simulink model "TutorialVariants"
settings: Solver=ode1  StartTime=0.0  StopTime=Inf  FixedStep=0.001  RelTol=1e-3
PostLoadFcn:
  | , if any(exist('dsrtsu_mdlpostloadfcn', 'file') == [2, 3, 6]), try dsrtsu_mdlpostloadfcn('Execute', bdroot); catch fprintf('Error in PostLoadFcn (dsrtsu_mdlpostloadfcn) for model "%s":\n %s\n', bdroot, lasterr); end, end,
undefined symbols (not defined in the file): rticanmm_blockfcn, rticanmm_initfcn
libraries: rtimmsu_dsrtlib x4
settings Model: RTICANMMDATA=struct('GeneralSetupData',struct('modelroot','E:\projects\dSPACE-RLS-Variants\current\RTICANMM\Components\Tutorial\Lesson10_results\RTICANMMTutorial_Lesson10','generalsettings',struct('filesettings',struct('destfolder',struct('Name','RTICANMM_FILES','Check',1),'buildfolder',struct('Name','.','Check',1),'AbsDestfolder',struct('Name','E:\projects\dSPACE-RLS-Variants\current\RTICANMM\Components\Tutorial\Lesson10_results\RTICANMMTutorial_Lesson10\RTICANMM_FILES'),'AbsBuildfolder',struct('Name','E:\projects\dSPACE-RLS-Variants\current\RTICANMM\Components\Tutorial\Lesson10_results\RTICANMMTutorial_Lesson10'))),'options',struct('addpaths',1,'rmpaths',1,'addtrcexclusion',logical(1),'cannavigator',struct('checkmonitoring',0,'checkinternmonitoring',1,'serviceno','31','hostservicedefheader',struct('name','RTICANMMHostService_TutorialVariants.h','path',['E:\CANMM_Tutorial\RLS2008-A\aus MKS\Lesson10_results\RTICANMMTutorial_Lesson10\RTICANMM_FILES\RTICANMMHostService_TutorialVariants.h'])),'show_usrtrc',0,'use_usrtrc',0,'addpath2usrmk',1),'advanced',struct('options',[1 1 1 1 1 1 1 1 1 1 1 1 1 1 1 1 1 1 1 1 1 1 1 1 1 1 1 1 1 1 1 1 1 1 1 1 1 1 1 1 1 1 1 1 1 1 1 1 1 1 1 1 1 1 1 1 1 1 1 1 1 1 1 1 1 1 1 1 1 1 1 1 1 1 1 1 1 1 1 1 1 1 1 1 1 1 1 1 1 1 1 1 1 1 1 1 1 1 1 1]),'MPSetup',{{}},'modelname','Lesson10_TutorialVariants','blockdata',struct('generalsettings',struct('filesettings',struct('destfolder',struct('Name','.','Check',1),'AbsDestfolder',struct('Name','T:\TOOL_SOURCES\CANnedy\m'),'buildfolder',struct('Name','.','Check',1),'AbsBuildfolder',struct('Name','C:\MATLAB6p5\work'))),'options',struct('addpaths',1,'rmpaths',1,'addpath2usrmk',1),'modelname','rticanmmlib','modelroot','T:\TOOL_SOURCES\CANnedy\m'),'userdata',struct('CANMMName',{{'TutVar_M1_V1','TutVar_M2','TutVar_M1_V2'}},'HostServiceChannelID',{{'TutVar_C1','TutVar_C2'}}),'RTI',struct('Type','RTI1005','Ver','7.1','Date','02-Nov-2013'),'version','3.0.735627.5512384259','MMType','RTICANMM','block',['Lesson10_TutorialVariants/RTICANMM' char(10) 'GeneralSetup']),'BuildData',struct('GeneralSetupData',struct('modelroot','D:\projects\dSPACE-RLS-Variants\current\RTICANMM\Components\Tutorial\Lesson10_results\RTICANMMTutorial_Lesson10','generalsettings',struct('filesettings',struct('destfolder',struct('Name','RTICANMM_FILES','Check',1),'buildfolder',struct('Name','.','Check',1),'AbsDestfolder',struct('Name','D:\projects\dSPACE-RLS-Variants\current\RTICANMM\Components\Tutorial\Lesson10_results\RTICANMMTutorial_Lesson10\RTICANMM_FILES'),'AbsBuildfolder',struct('Name','D:\projects\dSPACE-RLS-Variants\current\RTICANMM\Components\Tutorial\Lesson10_results\RTICANMMTutorial_Lesson10'))),'options',struct('addpaths',1,'rmpaths',1,'addtrcexclusion',logical(1),'cannavigator',struct('checkmonitoring',0,'checkinternmonitoring',1,'serviceno','31','hostservicedefheader',struct('name','RTICANMMHostService_TutorialVariants.h','path',['E:\CANMM_Tutorial\RLS2008-A\aus MKS\Lesson10_results\RTICANMMTutorial_Lesson10\RTICANMM_FILES\RTICANMMHostService_TutorialVariants.h'])),'show_usrtrc',0,'use_usrtrc',0,'addpath2usrmk',1),'advanced',struct('options',[1 1 1 1 1 1 1 1 1 1 1 1 1 1 1 1 1 1 1 1 1 1 1 1 1 1 1 1 1 1 1 1 1 1 1 1 1 1 1 1 1 1 1 1 1 1 1 1 1 1 1 1 1 1 1 1 1 1 1 1 1 1 1 1 1 1 1 1 1 1 1 1 1 1 1 1 1 1 1 1 1 1 1 1 1 1 1 1 1 1 1 1 1 1 1 1 1 1 1 1]),'MPSetup',{{}},'modelname','Lesson10_TutorialVariants','blockdata',struct('generalsettings',struct('filesettings',struct('destfolder',struct('Name','.','Check',1),'AbsDestfolder',struct('Name','T:\TOOL_SOURCES\CANnedy\m'),'buildfolder',struct('Name','.','Check',1),'AbsBuildfolder',struct('Name','C:\MATLAB6p5\work'))),'options',struct('addpaths',1,'rmpaths',1,'addpath2usrmk',1),'modelname','rticanmmlib','modelroot','T:\TOOL_SOURCES\CANnedy\m'),'userdata',struct('CANMMName',{{'TutVar_M1_V1','TutVar_M2','TutVar_M1_V2'}},'HostServiceChannelID',{{'TutVar_C1','TutVar_C2'}}),'RTI',struct('Type','RTI1005','Ver','6.6','Date','29-Nov-2010'),'version','2.5.4.734704.7639','MMType','RTICANMM','block',['Lesson10_TutorialVariants/RTICANMM' char(10) 'GeneralSetup']),'ModelBuildIsUpToDate',0))  RTILINMMDATA=struct('GeneralSetupData',[])  DSRTSU_INTERNAL_RTI_VER=430  DSRTSU_INTERNAL_RTI_TYPE=rti1005  DSRTSU_INTERNAL_RTIFLEXRAYCONFIG=60  DSRTSU_INTERNAL_RTIFPGA=30  BufferReuse=off  Creator=dSPACE GmbH  LastModifiedBy=dSPACE GmbH
settings DataIOCC: LimitDataPoints=on  SaveFormat=Array  SignalLoggingSaveFormat=ModelDataLogs  ReturnWorkspaceOutputs=off
settings OptimizationCC: BlockReduction=off  OptimizeBlockIOStorage=off  BufferReuse=off  ExpressionFolding=off  ExpressionDepthLimit=2147483647  LocalBlockOutputs=off  InitFltsAndDblsToZero=on  LifeSpan=inf  SimCompilerOptimization=Off
settings DebuggingCC: SaveWithParameterizedLinksMsg=none  UnderspecifiedInitializationDetection=Classic  MergeDetectMultiDrivingBlocksExec=none  SolverPrmCheckMsg=warning  MultiTaskCondExecSysMsg=none  FcnCallInpInsideContextMsg=Use local settings  FrameProcessingCompatibilityMsg=warning  StateNameClashWarn=warning  SFUnexpectedBacktrackingDiag=warning  SFNoUnconditionalDefaultTransitionDiag=warning
settings HardwareCC: ProdBitPerPointer=32  ProdLargestAtomicFloat=None  ProdEndianess=BigEndian  ProdWordSize=32  ProdHWDeviceType=Generic->Custom  TargetIntDivRoundTo=Zero  TargetEndianess=BigEndian  TargetHWDeviceType=Generic->Custom
settings ModelReferenceCC: PropagateSignalLabelsOutOfModel=off
settings SFSimCC: SimUseLocalCustomCode=off
settings RTWCC: SystemTargetFile=rti1005.tlc  MakeCommand=make_rti  TemplateMakefile=rti1005.tmf  Description=dSPACE DS1005 Hardware Platform  ProcessScript=rti1005_make_rtw_hook  RTWUseLocalCustomCode=off  IncludeERTFirstTime=on  RTWCompilerOptimization=Off
settings CodeAppCC: CustomSymbolStrType=$N$R$M
settings STFCustomTargetCC: TargetFcnLib=ansi_tfl_tmw.mat  CodeReplacementLibrary=ANSI_C  ParMdlRefBuildCompliant=on  GeneratePreprocessorConditionals=Disable all  SystemTargetFile=rti1005.tlc
settings GRTTargetCC: TargetFcnLib=ansi_tfl_tmw.mat  CodeReplacementLibrary=ANSI_C  CompOptLevelCompliant=off  ConcurrentExecutionCompliant=off  GeneratePreprocessorConditionals=Disable all  CombineOutputUpdateFcns=off  MatFileLogging=off  CPPClassGenCompliant=off  GRTInterface=on  ExtModeMexFile=noextcomm

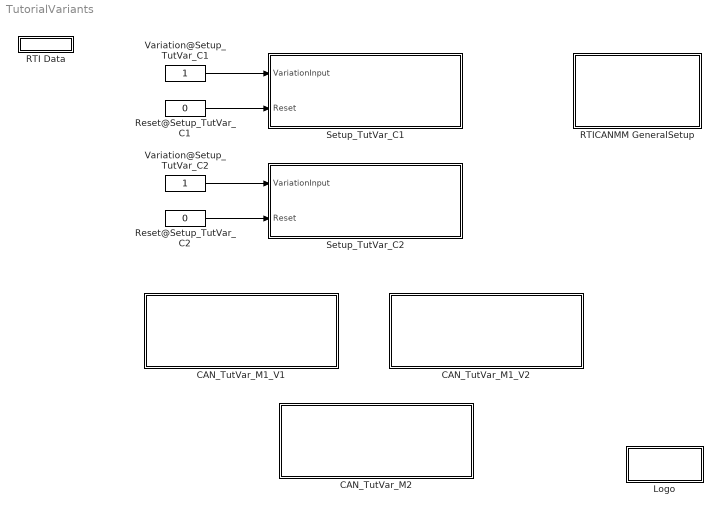
== system TutorialVariants ==
  CAN_TutVar_M1_V1 : Subsystem  InitFcn=rticanmm_blockfcn('InitFcn', 'CANnedy', gcb)  ClipboardFcn=rticanmm_blockfcn('ClipboardFcn', 'CANnedy', gcb)  mask(RTICANMM){DSProperties=struct('RTI',struct('Version',uint32(1),'BlockType',struct('isSLSource',uint8(1),'isSLSink',uint8(1),'isHWSource',uint8(0),'isHWSink',uint8(0),'isSetup',uint8(0),'isInline',uint8(1),'isNonInline',uint8(0),'isInterrupt',uint8(0),'isChannelwise',uint8(0)),'IOBoardType','RTICANMM','UnitType','RTICANMM','Identifier','Mainblock','DialogType','SL','BlockSet','RTICANMM','SlaveProcessor','CAN')), CANMMProperties=struct('RTICANMMVersion','3.0','RTICANMMVersionIntern','3.0.735627.5512384259','RTICANMMDate','02-May-2014','Settings','RTICANMM_MAIN_TutVar_M1_V1','UserTracePath','','ModelPath','E:\\projects\\dSPACE-RLS-Variants\\current\\RTICANMM\\Components\\Tutorial\\Lesson10_results\\RTICANMMTutorial_Lesson10','filesettings',struct('FileName','chassis.dbc','IsRelative',1,'ClusterId',1,'ClusterList',{{'default'}},'destfolder',struct('Name','RTICANMM_FILES','Check',1),'buildfolder',struct('Name','.','Check',1),'onlyfreerawcapture',0,'overlapping2variant',0),'onlyfreerawcapture',0,'Board','DS4302','BoardNum','1','ChannelNum','1','Variation','1','SetupId','TutVar_C1','MARK',['55E03A74395B53F8DB43BA9618B512';'A23C9334B1324361A95E8FCD407A20';'098F83A39FCF2835CF252EEA455F34';'6393CC0945E19D10F98F8B4C582B6C';'4BC1A51935C111E55014785F64462B'],'date','03-Feb-2014','clock',['03.02.2014 15:34:55'],'recreate',0,'RTIVER','RTI1005','j1939',0,'TRC',struct('include',1),'rtsupport',struct('XMLFile','E:\\projects\\dSPACE-RLS-Variants\\current\\RTICANMM\\Components\\Tutorial\\Lesson10_results\\RTICANMMTutorial_Lesson10\\RTICANMM_FILES\\RTICANMM_MAIN_TutVar_M1_V1.xml','DBCXML',struct('Path','E:\\projects\\dSPACE-RLS-Variants\\current\\RTICANMM\\Components\\Tutorial\\Lesson10_results\\RTICANMMTutorial_Lesson10\\RTICANMM_FILES\\RTICANMM_MAIN_TutVar_M1_V1_dbc.xml','support',1,'Name','chassis.dbc','Date',['09-Okt-2007 15:20:29'],'Type','mixed','DBCSupport','ON'))), CANMMType=CANnedy, CANMMUserTraceMerged=off, CANMMUserTracePath=, CANMMChannelNum=1, CANMMBoardNum=1, CANMMDestFolder=RTICANMM_FILES, CANMMFolder=., CANMMSetupId=TutVar_C1, CANMMsave2mat=['55E03A74395B53F8DB43BA9618B512';'A23C9334B1324361A95E8FCD407A20';'098F83A39FCF2835CF252EEA455F34';'6393CC0945E19D10F98F8B4C582B6C';'4BC1A51935C111E55014785F64462B'], CANMMName=TutVar_M1_V1, CANMMSettings=RTICANMM_MAIN_TutVar_M1_V1, CANMMIntermediateTag=RTICANMM_MAIN_TutVar_M1_V1_intermediate, CANMMsfcnname=RTICANMM_MAIN_TutVar_M1_V1}
      mask init:
      | rticanmm_initfcn(gcb, CANMMType, CANMMsfcnname)
      settings: AttributesFormatString=TutVar_C1[TutVar_M1_V1]: DS4302_B1_C1_V1  CopyFcn=rticanmm_blockfcn('CopyFcn', 'CANnedy', gcb)  DeleteFcn=rticanmm_blockfcn('DeleteFcn', 'CANnedy', gcb)  ModelCloseFcn=rticanmm_blockfcn('ModelCloseFcn', 'CANnedy', gcb)  NameChangeFcn=rticanmm_blockfcn('NameChangeFcn', 'CANnedy', gcb)  OpenFcn=try, rticanmm_main_gui('create',gcb); ; catch,errordlg({lasterr, '','Please check your RTI installation.'},['Error: ' upper(bdroot)], 'replace'); end  MoveFcn=rticanmm_blockfcn('MoveFcn', 'CANnedy', gcb)
      mask Help: eval('rticanmm_quickstart(''create'', gcb);', 'disp(lasterr);')
      mask Display: disp(sprintf('RTI CAN\nMultiMessage\nMainSetup'))
  CAN_TutVar_M1_V2 : Subsystem  InitFcn=rticanmm_blockfcn('InitFcn', 'CANnedy', gcb)  ClipboardFcn=rticanmm_blockfcn('ClipboardFcn', 'CANnedy', gcb)  mask(RTICANMM){DSProperties=struct('RTI',struct('Version',uint32(1),'BlockType',struct('isSLSource',uint8(1),'isSLSink',uint8(1),'isHWSource',uint8(0),'isHWSink',uint8(0),'isSetup',uint8(0),'isInline',uint8(1),'isNonInline',uint8(0),'isInterrupt',uint8(0),'isChannelwise',uint8(0)),'IOBoardType','RTICANMM','UnitType','RTICANMM','Identifier','Mainblock','DialogType','SL','BlockSet','RTICANMM','SlaveProcessor','CAN')), CANMMProperties=struct('RTICANMMVersion','3.0','RTICANMMVersionIntern','3.0.735627.5512384259','RTICANMMDate','02-May-2014','Settings','RTICANMM_MAIN_TutVar_M1_V2','UserTracePath','','ModelPath','E:\\projects\\dSPACE-RLS-Variants\\current\\RTICANMM\\Components\\Tutorial\\Lesson10_results\\RTICANMMTutorial_Lesson10','filesettings',struct('FileName','chassis_changed.dbc','IsRelative',1,'ClusterId',1,'ClusterList',{{'default'}},'destfolder',struct('Name','RTICANMM_FILES','Check',1),'buildfolder',struct('Name','.','Check',1),'onlyfreerawcapture',0,'overlapping2variant',0),'onlyfreerawcapture',0,'Board','DS4302','BoardNum','1','ChannelNum','1','Variation','2','SetupId','TutVar_C1','MARK',['7A753A0F068D0B04F07F060F8EC5AA';'9C128822ED17A9DECB1FCC6137CCCA';'527E1118F9B5998B502C4CF14A4AA0';'A533E42B0DF5453AD15DD1DE46811D';'0291723C433049D43F83E639655517'],'date','03-Feb-2014','clock',['03.02.2014 15:35:12'],'recreate',0,'RTIVER','RTI1005','j1939',0,'TRC',struct('include',1),'rtsupport',struct('XMLFile','E:\\projects\\dSPACE-RLS-Variants\\current\\RTICANMM\\Components\\Tutorial\\Lesson10_results\\RTICANMMTutorial_Lesson10\\RTICANMM_FILES\\RTICANMM_MAIN_TutVar_M1_V2.xml','DBCXML',struct('Path','E:\\projects\\dSPACE-RLS-Variants\\current\\RTICANMM\\Components\\Tutorial\\Lesson10_results\\RTICANMMTutorial_Lesson10\\RTICANMM_FILES\\RTICANMM_MAIN_TutVar_M1_V2_dbc.xml','support',1,'Name','chassis_changed.dbc','Date',['31-Mrz-2008 17:23:12'],'Type','mixed','DBCSupport','ON'))), CANMMType=CANnedy, CANMMUserTraceMerged=off, CANMMUserTracePath=, CANMMChannelNum=1, CANMMBoardNum=1, CANMMDestFolder=RTICANMM_FILES, CANMMFolder=., CANMMSetupId=TutVar_C1, CANMMsave2mat=['7A753A0F068D0B04F07F060F8EC5AA';'9C128822ED17A9DECB1FCC6137CCCA';'527E1118F9B5998B502C4CF14A4AA0';'A533E42B0DF5453AD15DD1DE46811D';'0291723C433049D43F83E639655517'], CANMMName=TutVar_M1_V2, CANMMSettings=RTICANMM_MAIN_TutVar_M1_V2, CANMMIntermediateTag=RTICANMM_MAIN_TutVar_M1_V2_intermediate, CANMMsfcnname=RTICANMM_MAIN_TutVar_M1_V2}
      mask init:
      | rticanmm_initfcn(gcb, CANMMType, CANMMsfcnname)
      settings: AttributesFormatString=TutVar_C1[TutVar_M1_V2]: DS4302_B1_C1_V2  CopyFcn=rticanmm_blockfcn('CopyFcn', 'CANnedy', gcb)  DeleteFcn=rticanmm_blockfcn('DeleteFcn', 'CANnedy', gcb)  ModelCloseFcn=rticanmm_blockfcn('ModelCloseFcn', 'CANnedy', gcb)  NameChangeFcn=rticanmm_blockfcn('NameChangeFcn', 'CANnedy', gcb)  OpenFcn=try, rticanmm_main_gui('create',gcb); ; catch,errordlg({lasterr, '','Please check your RTI installation.'},['Error: ' upper(bdroot)], 'replace'); end  MoveFcn=rticanmm_blockfcn('MoveFcn', 'CANnedy', gcb)
      mask Help: eval('rticanmm_quickstart(''create'', gcb);', 'disp(lasterr);')
      mask Display: disp(sprintf('RTI CAN\nMultiMessage\nMainSetup'))
  CAN_TutVar_M2 : Subsystem  InitFcn=rticanmm_blockfcn('InitFcn', 'CANnedy', gcb)  ClipboardFcn=rticanmm_blockfcn('ClipboardFcn', 'CANnedy', gcb)  mask(RTICANMM){DSProperties=struct('RTI',struct('Version',uint32(1),'BlockType',struct('isSLSource',uint8(1),'isSLSink',uint8(1),'isHWSource',uint8(0),'isHWSink',uint8(0),'isSetup',uint8(0),'isInline',uint8(1),'isNonInline',uint8(0),'isInterrupt',uint8(0),'isChannelwise',uint8(0)),'IOBoardType','RTICANMM','UnitType','RTICANMM','Identifier','Mainblock','DialogType','SL','BlockSet','RTICANMM','SlaveProcessor','CAN')), CANMMProperties=struct('RTICANMMVersion','3.0','RTICANMMVersionIntern','3.0.735627.5512384259','RTICANMMDate','02-May-2014','Settings','RTICANMM_MAIN_TutVar_M2','UserTracePath','','ModelPath','E:\\projects\\dSPACE-RLS-Variants\\current\\RTICANMM\\Components\\Tutorial\\Lesson10_results\\RTICANMMTutorial_Lesson10','filesettings',struct('FileName','','IsRelative',1,'ClusterId',1,'ClusterList',{{'default'}},'destfolder',struct('Name','RTICANMM_FILES','Check',1),'buildfolder',struct('Name','.','Check',1),'onlyfreerawcapture',1,'overlapping2variant',0),'onlyfreerawcapture',1,'Board','DS4302','BoardNum','1','ChannelNum','2','Variation','1','SetupId','TutVar_C2','MARK',['4BDFEA9EB9D32637AB0AA1F607449A';'11CDA3B00E5F6A73165C166F7F6289';'6163A90CBC928EA7712C5E92787D31';'7B56071945409C9EE63012215DB1F5';'8FDC3DAD5C2E7D1A171CC4627E2896'],'date','03-Feb-2014','clock',['03.02.2014 15:35:23'],'recreate',0,'RTIVER','RTI1005','j1939',0,'TRC',struct('include',1),'rtsupport',struct('XMLFile','E:\\projects\\dSPACE-RLS-Variants\\current\\RTICANMM\\Components\\Tutorial\\Lesson10_results\\RTICANMMTutorial_Lesson10\\RTICANMM_FILES\\RTICANMM_MAIN_TutVar_M2.xml','DBCXML',struct('Path','E:\\projects\\dSPACE-RLS-Variants\\current\\RTICANMM\\Components\\Tutorial\\Lesson10_results\\RTICANMMTutorial_Lesson10\\RTICANMM_FILES\\RTICANMM_MAIN_TutVar_M2_dbc.xml','support',0,'Name','','Date','','Type','','DBCSupport','OFF'))), CANMMType=CANnedy, CANMMUserTraceMerged=off, CANMMUserTracePath=, CANMMChannelNum=2, CANMMBoardNum=1, CANMMDestFolder=RTICANMM_FILES, CANMMFolder=., CANMMSetupId=TutVar_C2, CANMMsave2mat=['4BDFEA9EB9D32637AB0AA1F607449A';'11CDA3B00E5F6A73165C166F7F6289';'6163A90CBC928EA7712C5E92787D31';'7B56071945409C9EE63012215DB1F5';'8FDC3DAD5C2E7D1A171CC4627E2896'], CANMMName=TutVar_M2, CANMMSettings=RTICANMM_MAIN_TutVar_M2, CANMMIntermediateTag=RTICANMM_MAIN_TutVar_M2_intermediate, CANMMsfcnname=RTICANMM_MAIN_TutVar_M2}
      mask init:
      | rticanmm_initfcn(gcb, CANMMType, CANMMsfcnname)
      settings: AttributesFormatString=TutVar_C2[TutVar_M2]: DS4302_B1_C2_V1  CopyFcn=rticanmm_blockfcn('CopyFcn', 'CANnedy', gcb)  DeleteFcn=rticanmm_blockfcn('DeleteFcn', 'CANnedy', gcb)  ModelCloseFcn=rticanmm_blockfcn('ModelCloseFcn', 'CANnedy', gcb)  NameChangeFcn=rticanmm_blockfcn('NameChangeFcn', 'CANnedy', gcb)  OpenFcn=try, rticanmm_main_gui('create',gcb); ; catch,errordlg({lasterr, '','Please check your RTI installation.'},['Error: ' upper(bdroot)], 'replace'); end  MoveFcn=rticanmm_blockfcn('MoveFcn', 'CANnedy', gcb)
      mask Help: eval('rticanmm_quickstart(''create'', gcb);', 'disp(lasterr);')
      mask Display: disp(sprintf('RTI CAN\nMultiMessage\nMainSetup'))
  Logo : Subsystem  mask(dSPACE){EmptyParameter=[]}
      mask prompts: EmptyParameter "Mask Parameter 1:"
      settings: OpenFcn=;
      mask Display: image(imread('rti_lib_dslogo.tif'));
  RTI Data : Subsystem  Tag=struct('RTIDataServer',struct('RTIDataServerVs','2','RTIModelDescription','struct(''main'',''Lesson10_TutorialVariants'',''sub'',''Lesson10_TutorialVariants'',''isMp'',0)'))  LoadFcn="if exist('rtidc'), try,  rtidc('DataHostBlockClbLoad', gcbh); catch, disp(['Warning: ''LoadFcn'' for RTI Data block failed: ' lasterr]); end, end,"
      settings: CopyFcn="if exist('rtidc'), try,  rtidc('DataHostBlockClbCopy', gcbh); catch, disp(['Warning: ''CopyFcn'' for RTI Data block failed: ' lasterr]); end, end,"  DeleteFcn="if exist('rtidc'), try,  rtidc('DataHostBlockClbDelete', gcbh); catch, disp(['Warning: ''DeleteFcn'' for RTI Data block failed: ' lasterr]); end, end,"  ModelCloseFcn="if exist('rtidc'), try,  rtidc('DataHostBlockClbModelClose', gcbh); catch, disp(['Warning: ''ModelCloseFcn'' for RTI Data block failed: ' lasterr]); end, end,"  PreSaveFcn="if exist('rtidc'), try,  rtidc('DataHostBlockClbPreSave', gcbh); catch, disp(['Warning: ''PreSaveFcn'' for RTI Data block failed: ' lasterr]); end, end,"  PostSaveFcn="if exist('rtidc'), try,  rtidc('DataHostBlockClbPostSave', gcbh); catch, disp(['Warning: ''PostSaveFcn'' for RTI Data block failed: ' lasterr]); end, end,"  NameChangeFcn="if exist('rtidc'), try,  rtidc('DataHostBlockClbNameChange', gcbh); catch, disp(['Warning: ''NameChangeFcn'' for RTI Data block failed: ' lasterr]); end, end,"
      mask Type: RTI_DATA_HOST
      mask Description:
      | RTI Data Block.
      | This block is used by RTI to store internal model-dependent data.
      | Please keep this block on the root level of the model. Deleting this block will result in data loss.
      | 
      | NEVER DELETE OR COPY THIS BLOCK!
      mask Help:
      | RTI Data Block.
      | This block is used by RTI to store internal model-dependent data.
      | Please keep this block on the root level of the model. Deleting this block will result in data loss.
      | 
      | NEVER DELETE OR COPY THIS BLOCK!
      mask Display:
      | text(0.5, 0.5, 'RTI Data', 'HorizontalAlignment', 'center');
      | plot([1 0]);
  RTICANMM GeneralSetup : Subsystem  InitFcn=rticanmm_initfcn(gcb, 'CANnedySettings')  ClipboardFcn=rticanmm_blockfcn('ClipboardFcn', 'CANnedySettings', gcb)  mask(RTICANMM){DSProperties=struct('RTI',struct('Version',uint32(1),'BlockType',struct('isSLSource',uint8(1),'isSLSink',uint8(1),'isHWSource',uint8(0),'isHWSink',uint8(0),'isSetup',uint8(0),'isInline',uint8(1),'isNonInline',uint8(0),'isInterrupt',uint8(0),'isChannelwise',uint8(0)),'IOBoardType','RTICANMM','UnitType','RTICANMM','Identifier','GENERALSETUP','DialogType','SL','BlockSet','RTICANMM','SlaveProcessor','CAN')), CANMMDestFolder=RTICANMM_FILES, CANMMBuildDir=., CANMMAddPaths=on, CANMMAddpathUserMake=on, CANMMRemovePathOnclose=on, CANMMType=CANnedySettings, CANMMProperties=struct('modelroot','E:\\projects\\dSPACE-RLS-Variants\\current\\RTICANMM\\Components\\Tutorial\\Lesson10_results\\RTICANMMTutorial_Lesson10','generalsettings',struct('filesettings',struct('destfolder',struct('Name','RTICANMM_FILES','Check',1),'buildfolder',struct('Name','.','Check',1),'AbsDestfolder',struct('Name','E:\\projects\\dSPACE-RLS-Variants\\current\\RTICANMM\\Components\\Tutorial\\Lesson10_results\\RTICANMMTutorial_Lesson10\\RTICANMM_FILES'),'AbsBuildfolder',struct('Name','E:\\projects\\dSPACE-RLS-Variants\\current\\RTICANMM\\Components\\Tutorial\\Lesson10_results\\RTICANMMTutorial_Lesson10'))),'options',struct('addpaths',1,'rmpaths',1,'addtrcexclusion',logical(1),'cannavigator',struct('checkmonitoring',0,'checkinternmonitoring',1,'serviceno','31','hostservicedefheader',struct('name','RTICANMMHostService_TutorialVariants.h','path',['E:\\CANMM_Tutorial\\RLS2008-A\\aus MKS\\Lesson10_results\\RTICANMMTutorial_Lesson10\\RTICANMM_FILES\\RTICANMMHostService_TutorialVariants.h'])),'show_usrtrc',0,'use_usrtrc',0,'addpath2usrmk',1),'advanced',struct('options',[1 1 1 1 1 1 1 1 1 1 1 1 1 1 1 1 1 1 1 1 1 1 1 1 1 1 1 1 1 1 1 1 1 1 1 1 1 1 1 1 1 1 1 1 1 1 1 1 1 1 1 1 1 1 1 1 1 1 1 1 1 1 1 1 1 1 1 1 1 1 1 1 1 1 1 1 1 1 1 1 1 1 1 1 1 1 1 1 1 1 1 1 1 1 1 1 1 1 1 1]),'MPSetup',{{}},'modelname','Lesson10_TutorialVariants','blockdata',struct('generalsettings',struct('filesettings',struct('destfolder',struct('Name','.','Check',1),'AbsDestfolder',struct('Name','T:\\TOOL_SOURCES\\CANnedy\\m'),'buildfolder',struct('Name','.','Check',1),'AbsBuildfolder',struct('Name','C:\\MATLAB6p5\\work'))),'options',struct('addpaths',1,'rmpaths',1,'addpath2usrmk',1),'modelname','rticanmmlib','modelroot','T:\\TOOL_SOURCES\\CANnedy\\m'),'userdata',struct('CANMMName',{{'TutVar_M1_V1','TutVar_M2','TutVar_M1_V2'}},'HostServiceChannelID',{{'TutVar_C1','TutVar_C2'}}),'RTI',struct('Type','RTI1005','Ver','7.1','Date','02-Nov-2013'),'version','3.0.735627.5512384259','MMType','RTICANMM','block',['Lesson10_TutorialVariants/RTICANMM' char(10) 'GeneralSetup'])}
      mask prompts: CANMMDestFolder "Destination Folder for generated Files:"; CANMMBuildDir "Build Directory (*_usr.mk, *_usr.trc)"; CANMMAddPaths "Add Paths automatically"; CANMMAddpathUserMake "Add Paths to UserMake-File"; CANMMRemovePathOnclose "Remove added Path on ModelClose"
      mask init:
      | rticanmm_initfcn(gcb,'CANnedyGeneralSettings')
      settings: CopyFcn=rticanmm_blockfcn('CopyFcn', 'CANnedySettings', gcb)  DeleteFcn=rticanmm_blockfcn('DeleteFcn', 'CANnedySettings', gcb)  ModelCloseFcn=rticanmm_blockfcn('CloseFcn', 'CANnedyGeneralSettings', gcb)  NameChangeFcn=rticanmm_blockfcn('NameChangeFcn', 'CANnedySettings', gcb)  OpenFcn=try, rticanmm_gs_gui('create',gcb), ; catch,errordlg({lasterr, '','Please check your RTI installation.'},['Error: ' upper(bdroot)], 'replace'); end  MoveFcn=rticanmm_blockfcn('MoveFcn', 'CANnedySettings', gcb)
      mask Help: eval('rticanmm_quickstart(''create'', gcb);', 'disp(lasterr);')
      mask Display: disp(sprintf(['RTI CAN\nMultiMessage\nGeneralSetup']))
  Reset@Setup_TutVar_C1 : Constant  Value=0  OutDataTypeStr=boolean
  Reset@Setup_TutVar_C2 : Constant  Value=0  OutDataTypeStr=boolean
  Setup_TutVar_C1 : Subsystem  InitFcn=rticanmm_blockfcn('InitFcn', 'CANnedySetup', gcb)  ClipboardFcn=rticanmm_blockfcn('ClipboardFcn', 'CANnedySetup', gcb)  mask(RTICANMM){DSProperties=struct('RTI',struct('Version',uint32(1),'BlockType',struct('isSLSource',uint8(1),'isSLSink',uint8(1),'isHWSource',uint8(0),'isHWSink',uint8(0),'isSetup',uint8(0),'isInline',uint8(1),'isNonInline',uint8(0),'isInterrupt',uint8(0),'isChannelwise',uint8(0)),'IOBoardType','RTICANMM','UnitType','RTICANMM','Identifier','BUSSETUP','DialogType','SL','BlockSet','RTICANMM','SlaveProcessor','CAN')), CANMMProperties=struct('cannedy',struct('data',struct('options',struct('controllername','TutVar_C1','controllernameautomatic',0,'loglevel','0','checkrealtime',0,'checkchangebaudrate',0,'sampletime','1.000','CANControllerStatus',0,'NumberofStuffErr',0,'NumberofFormErr',0,'NumberofAckErr',0,'NumberofBit0Err',0,'NumberofsuccrecRX',0,'Numberofsuccsent',0,'NumberofBit1Err',0,'NumberofCRCErr',0,'NumberoflostRX',0,'Busoff',0,'Busload',0,'OperationPending',0,'TxRetryCount',3,'addtrcexclusion',logical(1),'cannavigator',struct('checkmonitoring',0,'checkinternmonitoring',0),'show_usrtrc',0,'use_usrtrc',0),'modelroot','E:\\CANMM_Tutorial\\RLS2008-A\\Lesson10_results\\RTICANMMTutorial_Lesson10','generalsettings',struct('setupdata',struct('board','DS4302','boardno',1,'channelno',1,'Type','STD','transceiver','ISO11898-2','busconfig','0x0','feedthrough','false','resistance',struct('r120',1,'roff',0,'r16',1,'r10',0),'baudrate','500','Frequency',[24 36],'samplemode',1,'commChannelTJA1041',6,'config',struct('standard',1,'advanced',0,'register',struct('btr0','0x40','btr1','0x1C','sp','87','sjw','1','tseg1','12','tseg2','1','brp','0','smpl','0','btr0_36','0x40','btr1_36','0x1C','sp_36','87','sjw_36','1','tseg1_36','12','tseg2_36','1','brp_36','0','smpl_36','0','btr0_64','0x40','btr1_64','0x1C','sp_64','87','sjw_64','1','tseg1_64','12','tseg2_64','1','brp_64','0','smpl_64','0')),'channelcfg',struct('INTENDISABLE','CAN_INT_DISABLE','intenable',0),'SETUPID','RTICANMM_TutVar_C1_ID','CONTROLLER_ID','CANMM_CTL_SETUP_TutVar_C1','mainblock_includefile','RTICANMM_SETUP_TutVar_C1','termination','TERMINATION_ON'),'filesettings',struct('destfolder',struct('Name','RTICANMM_FILES','Check',1),'buildfolder',struct('Name','.','Check',1))),'advanced',struct('options',[1 1 1 1 1 1 1 1 1 1 1 1 1 1 1 1 1 1 1 1 1 1 1 1 1 1 1 1 1 1 1 1 1 1 1 1 1 1 1 1 1 1 1 1 1 1 1 1 1 1 1 1 1 1 1 1 1 1 1 1 1 1 1 1 1 1 1 1 1 1 1 1 1 1 1 1 1 1 1 1 1 1 1 1 1 1 1 1 1 1 1 1 1 1 1 1 1 1 1 1]),'partialnetdata',struct('switchedon',0,'format','STD','idmask',['XXXXX XXXXXXXX XXXXXXXX XXXXXXXX'],'idcode','0','idfilter','0','datamaskused',0,'datalength','0','datamask','0x0000000000000000','partialnetworkenable',0)),'blk','Lesson10_TutorialVariants/Setup_TutVar_C1','allgeneratedfiles',{{'E:\\projects\\dSPACE-RLS-Variants\\current\\RTICANMM\\Components\\Tutorial\\Lesson10_results\\RTICANMMTutorial_Lesson10\\RTICANMM_FILES\\RTICANMM_SETUP_TutVar_C1.c','E:\\projects\\dSPACE-RLS-Variants\\current\\RTICANMM\\Components\\Tutorial\\Lesson10_results\\RTICANMMTutorial_Lesson10\\RTICANMM_FILES\\RTICANMM_SETUP_TutVar_C1.h','e:\\projects\\dspace-rls-variants\\current\\rticanmm\\components\\tutorial\\lesson10_results\\rticanmmtutorial_lesson10\\rticanmm_files\\rticanmm_setup_tutvar_c1.mexw32'}},'ismp',logical(0),'BlockDataVersion','0.6.0','recreate',0),'CANnedynew',0,'CANnedySettings','TutVar_C1','GeneratedFiles',{{'E:\\projects\\dSPACE-RLS-Variants\\current\\RTICANMM\\Components\\Tutorial\\Lesson10_results\\RTICANMMTutorial_Lesson10\\RTICANMM_FILES\\RTICANMM_SETUP_TutVar_C1.c','E:\\projects\\dSPACE-RLS-Variants\\current\\RTICANMM\\Components\\Tutorial\\Lesson10_results\\RTICANMMTutorial_Lesson10\\RTICANMM_FILES\\RTICANMM_SETUP_TutVar_C1.h','e:\\projects\\dspace-rls-variants\\current\\rticanmm\\components\\tutorial\\lesson10_results\\rticanmmtutorial_lesson10\\rticanmm_files\\rticanmm_setup_tutvar_c1.mexw32'}},'SFCN','RTICANMM_SETUP_TutVar_C1.c','HostService',struct('Tags',struct('DATA','RTICANMM_MonitorData','Enable','CANMMMonitor_TutVar_C1','TimeStamp','MonitoringTimeStamp_TutVar_C1'),'DATA',struct('Length',4),'Info',struct('Desc',{'ID','Service','Data1','Data2'}),'Names',struct('Enable','Monitoring_Enable','TimeStamp','Monitoring_TimeStamp'),'ChannelID',1)), CANMMType=CANnedySetup, CANMMFolder=E:\\projects\\dSPACE-RLS-Variants\\current\\RTICANMM\\Components\\Tutorial\\Lesson10_results\\RTICANMMTutorial_Lesson10, CANMMDestFolder=RTICANMM_FILES, CANMMSettings=TutVar_C1, CANMMSFcn=RTICANMM_SETUP_TutVar_C1, CANMMBoard=DS4302, CANMMBoardNum=1, CANMMChannel=1}
      settings: AttributesFormatString=%<CANMMSettings>: %<CANMMBoard>_B%<CANMMBoardNum>_C%<CANMMChannel>  CopyFcn=rticanmm_blockfcn('CopyFcn', 'CANnedySetup', gcb)  DeleteFcn=rticanmm_blockfcn('DeleteFcn', 'CANnedySetup', gcb)  ModelCloseFcn=rticanmm_blockfcn('ModelCloseFcn', 'CANnedySetup', gcb)  NameChangeFcn=rticanmm_blockfcn('NameChangeFcn', 'CANnedySetup', gcb)  OpenFcn=try, rticanmm_setup_gui('create',gcb); ; catch,errordlg({lasterr, '','Please check your RTI installation.'},['Error: ' upper(bdroot)], 'replace'); end  MoveFcn=rticanmm_blockfcn('MoveFcn', 'CANnedySetup', gcb)
      mask Help: eval('rticanmm_quickstart(''create'', gcb);', 'disp(lasterr);')
      mask Display:
      | disp('RTI CAN\nMultiMessage\nControllerSetup')
      | 
      | port_label('input', 1 , 'Variation')
      | port_label('input', 2 , 'Reset')
  Setup_TutVar_C2 : Subsystem  InitFcn=rticanmm_blockfcn('InitFcn', 'CANnedySetup', gcb)  ClipboardFcn=rticanmm_blockfcn('ClipboardFcn', 'CANnedySetup', gcb)  mask(RTICANMM){DSProperties=struct('RTI',struct('Version',uint32(1),'BlockType',struct('isSLSource',uint8(1),'isSLSink',uint8(1),'isHWSource',uint8(0),'isHWSink',uint8(0),'isSetup',uint8(0),'isInline',uint8(1),'isNonInline',uint8(0),'isInterrupt',uint8(0),'isChannelwise',uint8(0)),'IOBoardType','RTICANMM','UnitType','RTICANMM','Identifier','BUSSETUP','DialogType','SL','BlockSet','RTICANMM','SlaveProcessor','CAN')), CANMMProperties=struct('cannedy',struct('data',struct('options',struct('controllername','TutVar_C2','controllernameautomatic',0,'loglevel','0','checkrealtime',0,'checkchangebaudrate',0,'sampletime','1.000','CANControllerStatus',0,'NumberofStuffErr',0,'NumberofFormErr',0,'NumberofAckErr',0,'NumberofBit0Err',0,'NumberofsuccrecRX',0,'Numberofsuccsent',0,'NumberofBit1Err',0,'NumberofCRCErr',0,'NumberoflostRX',0,'Busoff',0,'Busload',0,'OperationPending',0,'TxRetryCount',3,'addtrcexclusion',logical(1),'cannavigator',struct('checkmonitoring',0,'checkinternmonitoring',0),'show_usrtrc',0,'use_usrtrc',0),'modelroot','E:\\CANMM_Tutorial\\RLS2008-A\\Lesson10_results\\RTICANMMTutorial_Lesson10','generalsettings',struct('setupdata',struct('board','DS4302','boardno',1,'channelno',2,'Type','STD','transceiver','ISO11898-2','busconfig','0x0','feedthrough','false','resistance',struct('r120',1,'roff',0,'r16',1,'r10',0),'baudrate','500','Frequency',[24 36],'samplemode',1,'commChannelTJA1041',6,'config',struct('standard',1,'advanced',0,'register',struct('btr0','0x40','btr1','0x1C','sp','87','sjw','1','tseg1','12','tseg2','1','brp','0','smpl','0','btr0_36','0x40','btr1_36','0x1C','sp_36','87','sjw_36','1','tseg1_36','12','tseg2_36','1','brp_36','0','smpl_36','0','btr0_64','0x40','btr1_64','0x1C','sp_64','87','sjw_64','1','tseg1_64','12','tseg2_64','1','brp_64','0','smpl_64','0')),'channelcfg',struct('INTENDISABLE','CAN_INT_DISABLE','intenable',0),'SETUPID','RTICANMM_TutVar_C2_ID','CONTROLLER_ID','CANMM_CTL_SETUP_TutVar_C2','mainblock_includefile','RTICANMM_SETUP_TutVar_C2','termination','TERMINATION_ON'),'filesettings',struct('destfolder',struct('Name','RTICANMM_FILES','Check',1),'buildfolder',struct('Name','.','Check',1))),'advanced',struct('options',[1 1 1 1 1 1 1 1 1 1 1 1 1 1 1 1 1 1 1 1 1 1 1 1 1 1 1 1 1 1 1 1 1 1 1 1 1 1 1 1 1 1 1 1 1 1 1 1 1 1 1 1 1 1 1 1 1 1 1 1 1 1 1 1 1 1 1 1 1 1 1 1 1 1 1 1 1 1 1 1 1 1 1 1 1 1 1 1 1 1 1 1 1 1 1 1 1 1 1 1]),'partialnetdata',struct('switchedon',0,'format','STD','idmask',['XXXXX XXXXXXXX XXXXXXXX XXXXXXXX'],'idcode','0','idfilter','0','datamaskused',0,'datalength','0','datamask','0x0000000000000000','partialnetworkenable',0)),'blk','Lesson10_TutorialVariants/Setup_TutVar_C2','allgeneratedfiles',{{'E:\\projects\\dSPACE-RLS-Variants\\current\\RTICANMM\\Components\\Tutorial\\Lesson10_results\\RTICANMMTutorial_Lesson10\\RTICANMM_FILES\\RTICANMM_SETUP_TutVar_C2.c','E:\\projects\\dSPACE-RLS-Variants\\current\\RTICANMM\\Components\\Tutorial\\Lesson10_results\\RTICANMMTutorial_Lesson10\\RTICANMM_FILES\\RTICANMM_SETUP_TutVar_C2.h','e:\\projects\\dspace-rls-variants\\current\\rticanmm\\components\\tutorial\\lesson10_results\\rticanmmtutorial_lesson10\\rticanmm_files\\rticanmm_setup_tutvar_c2.mexw32'}},'ismp',logical(0),'BlockDataVersion','0.6.0','recreate',0),'CANnedynew',0,'CANnedySettings','TutVar_C2','GeneratedFiles',{{'E:\\projects\\dSPACE-RLS-Variants\\current\\RTICANMM\\Components\\Tutorial\\Lesson10_results\\RTICANMMTutorial_Lesson10\\RTICANMM_FILES\\RTICANMM_SETUP_TutVar_C2.c','E:\\projects\\dSPACE-RLS-Variants\\current\\RTICANMM\\Components\\Tutorial\\Lesson10_results\\RTICANMMTutorial_Lesson10\\RTICANMM_FILES\\RTICANMM_SETUP_TutVar_C2.h','e:\\projects\\dspace-rls-variants\\current\\rticanmm\\components\\tutorial\\lesson10_results\\rticanmmtutorial_lesson10\\rticanmm_files\\rticanmm_setup_tutvar_c2.mexw32'}},'SFCN','RTICANMM_SETUP_TutVar_C2.c','HostService',struct('Tags',struct('DATA','RTICANMM_MonitorData','Enable','CANMMMonitor_TutVar_C2','TimeStamp','MonitoringTimeStamp_TutVar_C2'),'DATA',struct('Length',4),'Info',struct('Desc',{'ID','Service','Data1','Data2'}),'Names',struct('Enable','Monitoring_Enable','TimeStamp','Monitoring_TimeStamp'),'ChannelID',2)), CANMMType=CANnedySetup, CANMMFolder=E:\\projects\\dSPACE-RLS-Variants\\current\\RTICANMM\\Components\\Tutorial\\Lesson10_results\\RTICANMMTutorial_Lesson10, CANMMDestFolder=RTICANMM_FILES, CANMMSettings=TutVar_C2, CANMMSFcn=RTICANMM_SETUP_TutVar_C2, CANMMBoard=DS4302, CANMMBoardNum=1, CANMMChannel=2}
      settings: AttributesFormatString=%<CANMMSettings>: %<CANMMBoard>_B%<CANMMBoardNum>_C%<CANMMChannel>  CopyFcn=rticanmm_blockfcn('CopyFcn', 'CANnedySetup', gcb)  DeleteFcn=rticanmm_blockfcn('DeleteFcn', 'CANnedySetup', gcb)  ModelCloseFcn=rticanmm_blockfcn('ModelCloseFcn', 'CANnedySetup', gcb)  NameChangeFcn=rticanmm_blockfcn('NameChangeFcn', 'CANnedySetup', gcb)  OpenFcn=try, rticanmm_setup_gui('create',gcb); ; catch,errordlg({lasterr, '','Please check your RTI installation.'},['Error: ' upper(bdroot)], 'replace'); end  MoveFcn=rticanmm_blockfcn('MoveFcn', 'CANnedySetup', gcb)
      mask Help: eval('rticanmm_quickstart(''create'', gcb);', 'disp(lasterr);')
      mask Display:
      | disp('RTI CAN\nMultiMessage\nControllerSetup')
      | 
      | port_label('input', 1 , 'Variation')
      | port_label('input', 2 , 'Reset')
  Variation@Setup_TutVar_C1 : Constant  OutDataTypeStr=uint8
  Variation@Setup_TutVar_C2 : Constant  OutDataTypeStr=uint8
  wires:
  Variation@Setup_TutVar_C1/1 -> Setup_TutVar_C1/1(VariationInput)
  Reset@Setup_TutVar_C1/1 -> Setup_TutVar_C1/2(Reset)
  Variation@Setup_TutVar_C2/1 -> Setup_TutVar_C2/1(VariationInput)
  Reset@Setup_TutVar_C2/1 -> Setup_TutVar_C2/2(Reset)

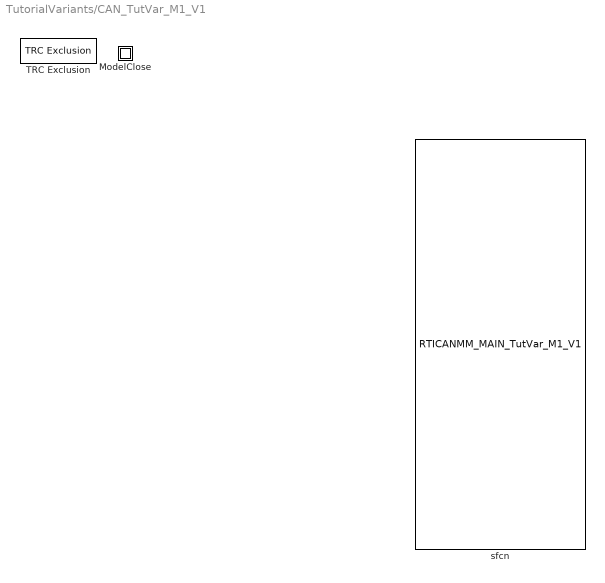
== system TutorialVariants/CAN_TutVar_M1_V1 ==
  ModelClose : Subsystem
      mask Type: RTICANMMModelClose
  TRC Exclusion : rtimmsu_dsrtlib/TRC Exclusion
  sfcn : S-Function  InitFcn=rticanmm_initfcn(gcb, 'SFCNs')  FunctionName=RTICANMM_MAIN_TutVar_M1_V1  EnableBusSupport=off
      mask init:
      | rticanmm_initfcn(gcb, 'SFCNs')

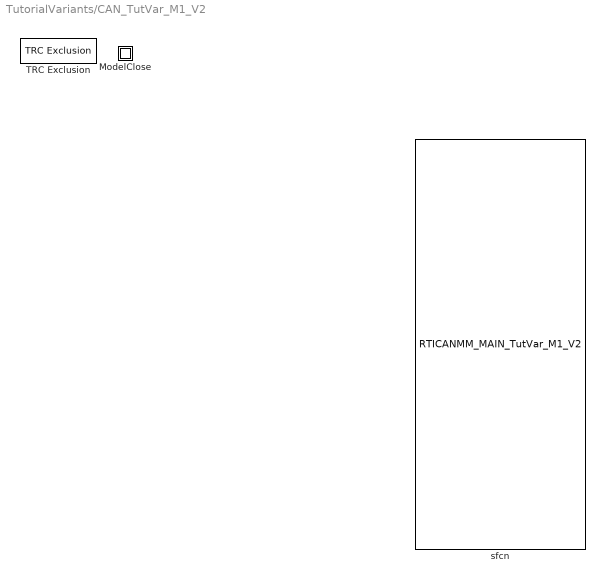
== system TutorialVariants/CAN_TutVar_M1_V2 ==
  ModelClose : Subsystem
      mask Type: RTICANMMModelClose
  TRC Exclusion : rtimmsu_dsrtlib/TRC Exclusion
  sfcn : S-Function  InitFcn=rticanmm_initfcn(gcb, 'SFCNs')  FunctionName=RTICANMM_MAIN_TutVar_M1_V2  EnableBusSupport=off
      mask init:
      | rticanmm_initfcn(gcb, 'SFCNs')

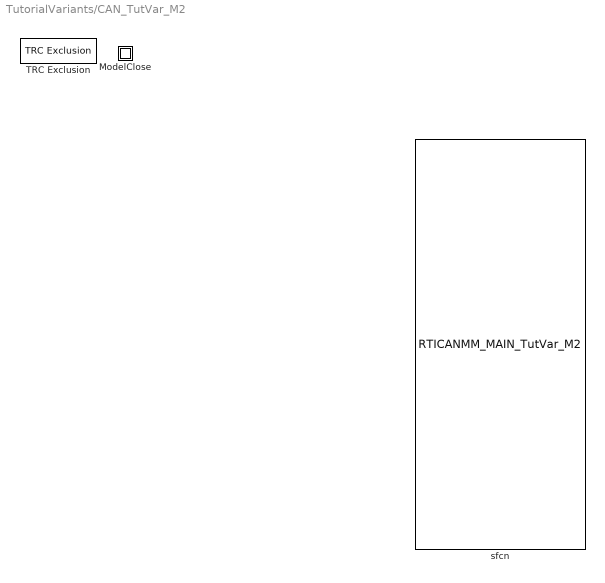
== system TutorialVariants/CAN_TutVar_M2 ==
  ModelClose : Subsystem
      mask Type: RTICANMMModelClose
  TRC Exclusion : rtimmsu_dsrtlib/TRC Exclusion
  sfcn : S-Function  InitFcn=rticanmm_initfcn(gcb, 'SFCNs')  FunctionName=RTICANMM_MAIN_TutVar_M2  EnableBusSupport=off
      mask init:
      | rticanmm_initfcn(gcb, 'SFCNs')

== system TutorialVariants/Logo ==
  note: $RCSfile: Lesson10_TutorialVariants.mdl $
  note: $Date: 2013/07/08 14:43:11MESZ $
  note: $Revision: 1.12 $

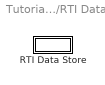
== system TutorialVariants/RTI Data ==
  RTI Data Store : Subsystem  Tag=struct('private',struct('version',struct('dsVer',uint32(2)),'access',struct('modified',['03-Feb-2014 15:35:24'],'type','Model','isPerm',1)),'public',struct('main',struct('data',[]),'sub',struct('name','','data',[])))
      mask Type: RTI_DATA_STORE
      mask Description:
      | RTI Data Store Block. This block is used by RTI to store internal model dependent data. Deleting this block will result in data loss.
      | 
      | NEVER DELETE, COPY, OR MODIFY THIS BLOCK!
      mask Help:
      | RTI Data Store Block. This block is used by RTI to store internal model dependent data. Deleting this block will result in data loss.
      | 
      | NEVER DELETE, COPY, OR MODIFY THIS BLOCK!
      mask Display: text(0.5, 0.5, ' ', 'HorizontalAlignment', 'center');

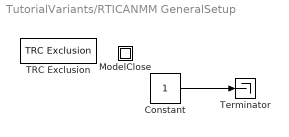
== system TutorialVariants/RTICANMM GeneralSetup ==
  Constant : Constant
  ModelClose : Subsystem
      mask Type: RTICANMMModelClose
  TRC Exclusion : rtimmsu_dsrtlib/TRC Exclusion
  Terminator : Terminator
  wires:
  Constant/1 -> Terminator/1

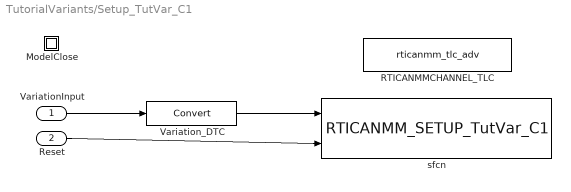
== system TutorialVariants/Setup_TutVar_C1 ==
  VariationInput : Inport
  Reset : Inport  Port=2
  ModelClose : Subsystem
      mask Type: RTICANMMModelClose
  RTICANMMCHANNEL_TLC : S-Function  FunctionName=rticanmm_tlc_adv  Parameters=4302,1,1,0,500,'unused'  EnableBusSupport=off
      mask Type: RTICANMMCHANNEL_TLC
  Variation_DTC : DataTypeConversion  SaturateOnIntegerOverflow=on  RndMeth=Zero
  sfcn : S-Function  InitFcn=rticanmm_initfcn(gcb, 'SFCNs')  FunctionName=RTICANMM_SETUP_TutVar_C1  EnableBusSupport=off
      mask init:
      | rticanmm_initfcn(gcb, 'SFCNs')
  wires:
  Reset/1 -> sfcn/2
  VariationInput/1 -> Variation_DTC/1
  Variation_DTC/1 -> sfcn/1

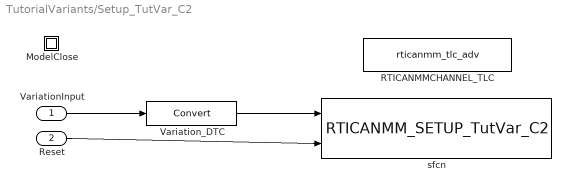
== system TutorialVariants/Setup_TutVar_C2 ==
  VariationInput : Inport
  Reset : Inport  Port=2
  ModelClose : Subsystem
      mask Type: RTICANMMModelClose
  RTICANMMCHANNEL_TLC : S-Function  FunctionName=rticanmm_tlc_adv  Parameters=4302,1,2,0,500,'unused'  EnableBusSupport=off
      mask Type: RTICANMMCHANNEL_TLC
  Variation_DTC : DataTypeConversion  SaturateOnIntegerOverflow=on  RndMeth=Zero
  sfcn : S-Function  InitFcn=rticanmm_initfcn(gcb, 'SFCNs')  FunctionName=RTICANMM_SETUP_TutVar_C2  EnableBusSupport=off
      mask init:
      | rticanmm_initfcn(gcb, 'SFCNs')
  wires:
  Reset/1 -> sfcn/2
  VariationInput/1 -> Variation_DTC/1
  Variation_DTC/1 -> sfcn/1

== system TutorialVariants/CAN_TutVar_M1_V1/ModelClose ==

== system TutorialVariants/CAN_TutVar_M1_V2/ModelClose ==

== system TutorialVariants/CAN_TutVar_M2/ModelClose ==

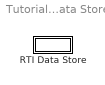
== system TutorialVariants/RTI Data/RTI Data Store ==
  RTI Data Store : Subsystem
      mask Type: RTI_DATA_STORE
      mask Description:
      | RTI Data Store Block. This block is used by RTI to store internal model dependent data. Deleting this block will result in data loss.
      | 
      | NEVER DELETE, COPY, OR MODIFY THIS BLOCK!
      mask Help:
      | RTI Data Store Block. This block is used by RTI to store internal model dependent data. Deleting this block will result in data loss.
      | 
      | NEVER DELETE, COPY, OR MODIFY THIS BLOCK!
      mask Display: text(0.5, 0.5, ' ', 'HorizontalAlignment', 'center');

== system TutorialVariants/RTICANMM GeneralSetup/ModelClose ==

== system TutorialVariants/Setup_TutVar_C1/ModelClose ==

== system TutorialVariants/Setup_TutVar_C2/ModelClose ==

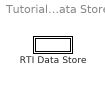
== system TutorialVariants/RTI Data/RTI Data Store/RTI Data Store ==
  RTI Data Store : Subsystem
      mask Type: RTI_DATA_STORE
      mask Description:
      | RTI Data Store Block. This block is used by RTI to store internal model dependent data. Deleting this block will result in data loss.
      | 
      | NEVER DELETE, COPY, OR MODIFY THIS BLOCK!
      mask Help:
      | RTI Data Store Block. This block is used by RTI to store internal model dependent data. Deleting this block will result in data loss.
      | 
      | NEVER DELETE, COPY, OR MODIFY THIS BLOCK!
      mask Display: text(0.5, 0.5, ' ', 'HorizontalAlignment', 'center');

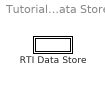
== system TutorialVariants/RTI Data/RTI Data Store/RTI Data Store/RTI Data Store ==
  RTI Data Store : Subsystem
      mask Type: RTI_DATA_STORE
      mask Description:
      | RTI Data Store Block. This block is used by RTI to store internal model dependent data. Deleting this block will result in data loss.
      | 
      | NEVER DELETE, COPY, OR MODIFY THIS BLOCK!
      mask Help:
      | RTI Data Store Block. This block is used by RTI to store internal model dependent data. Deleting this block will result in data loss.
      | 
      | NEVER DELETE, COPY, OR MODIFY THIS BLOCK!
      mask Display: text(0.5, 0.5, ' ', 'HorizontalAlignment', 'center');

== system TutorialVariants/RTI Data/RTI Data Store/RTI Data Store/RTI Data Store/RTI Data Store ==
